simulink model "model_induction_Motor_V_F_Control_v2"  (R2017b)
settings: Solver=ode23s  StartTime=0.0  StopTime=10.0  MaxStep=1e-4  RelTol=1e-3
libraries: powerlib x20, simulink x9
settings Model: SimulationMode=accelerator  Creator=proso  LastModifiedBy=proso
settings OptimizationCC: EfficientMapNaN2IntZero=off
settings HardwareCC: TargetBitPerPointer=64  TargetBitPerSizeT=64  TargetBitPerPtrDiffT=64  TargetLongLongMode=on  TargetIntDivRoundTo=Zero  TargetEndianess=LittleEndian  TargetWordSize=64  TargetHWDeviceType=MATLAB Host  ProdEqTarget=off
settings CodeAppCC: MaxIdLength=128
settings GRTTargetCC: TargetLangStandard=C89/C90 (ANSI)  CombineOutputUpdateFcns=off  GRTInterface=on

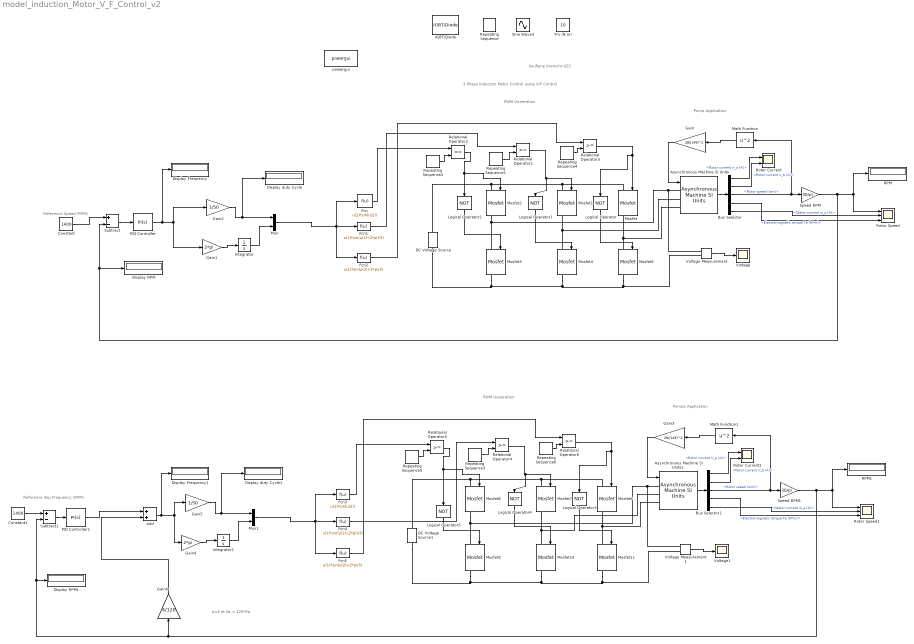
== system model_induction_Motor_V_F_Control_v2 ==
  note: p=4 et Ns = 120*f/p
  note: Reference Speed (RPM)
  note: Pump Application
  note: PWM Generation
  note: 3 Phase Induction Motor Control using V/F Control
  note: Soufiane Kremcht GE2
  note: PWM Generation
  note: Reference Slip Frequency (RPM)
  note: Pompe Application
  Add : Sum
  Asynchronous Machine SI Units : powerlib/Machines/Asynchronous Machine SI Units  RotorType=Squirrel-cage  PresetModel="15:  5.4 HP (4KW)   400 V  50Hz 1430 RPM"  MechanicalLoad=Torque Tm  ShowDetailedParameters=on  ReferenceFrame=Rotor  Units=SI  MeasurementBus=off  NominalParameters=[4000 400 50]  Stator=[1.405 0.005839]  Rotor=[1.395 0.005839]  Cage1=[1.543 0.006067]  Cage2=[3.309 0.005654]  Lm=0.1722  Mechanical=[0.0131 0.002985 2]  PolePairs=2  InitialConditions=[1 0 0 0 0 0 0 0]  SimulateSaturation=off  Saturation=[14.03593122, 27.81365428, 53.79336849, 72.68890987, 97.98006896, 148.6815601, 215.7428561, 302.9841135, 428.7778367 ; 230, 322, 414, 460, 506, 552, 598, 644, 690]  LoadFlowParameters=1492000  TsPowergui=0  TsBlock=-1  IterativeModel=Trapezoidal non iterative  IterativeDiscreteModel=Trapezoidal non iterative  Pmec=1.492e+006
  Asynchronous Machine SI Units1 : powerlib/Machines/Asynchronous Machine SI Units  RotorType=Squirrel-cage  PresetModel="15:  5.4 HP (4KW)   400 V  50Hz 1430 RPM"  MechanicalLoad=Torque Tm  ShowDetailedParameters=on  ReferenceFrame=Rotor  Units=SI  MeasurementBus=off  NominalParameters=[4000 400 50]  Stator=[1.405 0.005839]  Rotor=[1.395 0.005839]  Cage1=[1.543 0.006067]  Cage2=[3.309 0.005654]  Lm=0.1722  Mechanical=[0.0131 0.002985 2]  PolePairs=2  InitialConditions=[1 0 0 0 0 0 0 0]  SimulateSaturation=off  Saturation=[14.03593122, 27.81365428, 53.79336849, 72.68890987, 97.98006896, 148.6815601, 215.7428561, 302.9841135, 428.7778367 ; 230, 322, 414, 460, 506, 552, 598, 644, 690]  LoadFlowParameters=1492000  TsPowergui=0  TsBlock=-1  IterativeModel=Trapezoidal non iterative  IterativeDiscreteModel=Trapezoidal non iterative  Pmec=1.492e+006
  Bus Selector : BusSelector  OutputSignals=Rotor measurements.Rotor current ir_a (A),Rotor measurements.Rotor current ir_b (A),Mechanical.Rotor speed (wm),Mechanical.Electromagnetic torque Te (N*m),Stator measurements.Stator current is_a (A)
  Bus Selector1 : BusSelector  OutputSignals=Rotor measurements.Rotor current ir_a (A),Rotor measurements.Rotor current ir_b (A),Mechanical.Rotor speed (wm),Mechanical.Electromagnetic torque Te (N*m),Stator measurements.Stator current is_a (A)
  Constant : Constant  Value=1400
  Constant1 : Constant  Value=1400
  DC Voltage Source : powerlib/Electrical Sources/DC Voltage Source  Amplitude=650  Measurements=None
  DC Voltage Source1 : powerlib/Electrical Sources/DC Voltage Source  Amplitude=650  Measurements=None
  Display Frequency : Display
  Display Frequency1 : Display
  Display RPM : Display
  Display RPM1 : Display
  Display duty Cycle : Display
  Display duty Cycle1 : Display
  Fcn : Fcn  Expr=u(1)*sin(u(2))
  Fcn1 : Fcn  Expr=u(1)*sin(u(2)-(2*pi)/3)
  Fcn2 : Fcn  Expr=u(1)*sin(u(2)+2*pi/3)
  Fcn3 : Fcn  Expr=u(1)*sin(u(2))
  Fcn4 : Fcn  Expr=u(1)*sin(u(2)-(2*pi)/3)
  Fcn5 : Fcn  Expr=u(1)*sin(u(2)+2*pi/3)
  Gain : Gain  Gain=28/(149)^2
  Gain1 : Gain  Gain=2*pi
  Gain2 : Gain  Gain=1/50
  Gain3 : Gain  Gain=28/(149)^2
  Gain4 : Gain  Gain=2*pi
  Gain5 : Gain  Gain=1/50
  Gain6 : Gain  Gain=4/120
  IGBT/Diode : powerlib/Power Electronics/IGBT//Diode  Ron=1e-3  Rs=1e5  Cs=inf  Measurements=on
  Integrator : Integrator
  Integrator1 : Integrator
  Logical Operator{,1..5} (6 alike) : Logic  Operator=NOT  AllPortsSameDT=off  OutDataTypeStr=boolean
  Math Function : Math  Operator=square  SaturateOnIntegerOverflow=on
  Math Function1 : Math  Operator=square  SaturateOnIntegerOverflow=on
  Mosfet{,1..11} (12 alike) : powerlib/Power Electronics/Mosfet  Ron=0.1  Lon=0  Rd=0.01  Vfd=0  IC=0  Rs=1e5  Cs=inf  Measurements=on
  Mux : Mux  Inputs=2
  Mux1 : Mux  Inputs=2
  PID Controller : simulink/Continuous/PID Controller  Controller=PI  TimeDomain=Continuous-time  SampleTime=-1  IntegratorMethod=Forward Euler  FilterMethod=Forward Euler  Form=Parallel  UseFilter=on  ControllerParametersSource=internal  P=0.001  I=0.1  D=0  N=100  InitialConditionSource=internal  InitialConditionForIntegrator=0  InitialConditionForFilter=0  ExternalReset=none  LimitOutput=on  UpperSaturationLimit=50  LowerSaturationLimit=-50  LinearizeAsGain=on  AntiWindupMode=clamping  Kb=1  TrackingMode=off  Kt=1  PParamMin=[]  PParamMax=[]  IParamMin=[]  IParamMax=[]  DParamMin=[]  DParamMax=[]  NParamMin=[]  NParamMax=[]  KbParamMin=[]  KbParamMax=[]  KtParamMin=[]  KtParamMax=[]  POutMin=[]  POutMax=[]  IOutMin=[]  IOutMax=[]  DOutMin=[]  DOutMax=[]  NOutMin=[]  NOutMax=[]  KbOutMin=[]  KbOutMax=[]  KtOutMin=[]  KtOutMax=[]  IntegratorOutMin=[]  IntegratorOutMax=[]  FilterOutMin=[]  FilterOutMax=[]  SumOutMin=[]  SumOutMax=[]  SumI1OutMin=[]  SumI1OutMax=[]  SumI2OutMin=[]  SumI2OutMax=[]  SumI3OutMin=[]  SumI3OutMax=[]  SumDOutMin=[]  SumDOutMax=[]  SaturationOutMin=[]  SaturationOutMax=[]  IntegratorContinuousStateAttributes=''  IntegratorStateMustResolveToSignalObject=off  IntegratorRTWStateStorageClass=Auto  FilterContinuousStateAttributes=''  FilterStateMustResolveToSignalObject=off  FilterRTWStateStorageClass=Auto  DifferentiatorICPrevScaledInput=0  DifferentiatorOutMin=[]  DifferentiatorOutMax=[]  InitialConditionSetting=State (most efficient)  FilterDiffOutCoefMin=[]  FilterDiffOutCoefMax=[]  SumDenOutMin=[]  SumDenOutMax=[]  SumNumOutMin=[]  SumNumOutMax=[]  ReciprocalOutMin=[]  ReciprocalOutMax=[]  DivideOutMin=[]  DivideOutMax=[]  TunerSelectOption=Transfer Function Based (PID Tuner App)
  PID Controller1 : simulink/Continuous/PID Controller  Controller=PI  TimeDomain=Continuous-time  SampleTime=-1  IntegratorMethod=Forward Euler  FilterMethod=Forward Euler  Form=Parallel  UseFilter=on  ControllerParametersSource=internal  P=1.5  I=0.01  D=0  N=100  InitialConditionSource=internal  InitialConditionForIntegrator=0  InitialConditionForFilter=0  ExternalReset=none  LimitOutput=on  UpperSaturationLimit=50  LowerSaturationLimit=-50  LinearizeAsGain=on  AntiWindupMode=clamping  Kb=1  TrackingMode=off  Kt=1  PParamMin=[]  PParamMax=[]  IParamMin=[]  IParamMax=[]  DParamMin=[]  DParamMax=[]  NParamMin=[]  NParamMax=[]  KbParamMin=[]  KbParamMax=[]  KtParamMin=[]  KtParamMax=[]  POutMin=[]  POutMax=[]  IOutMin=[]  IOutMax=[]  DOutMin=[]  DOutMax=[]  NOutMin=[]  NOutMax=[]  KbOutMin=[]  KbOutMax=[]  KtOutMin=[]  KtOutMax=[]  IntegratorOutMin=[]  IntegratorOutMax=[]  FilterOutMin=[]  FilterOutMax=[]  SumOutMin=[]  SumOutMax=[]  SumI1OutMin=[]  SumI1OutMax=[]  SumI2OutMin=[]  SumI2OutMax=[]  SumI3OutMin=[]  SumI3OutMax=[]  SumDOutMin=[]  SumDOutMax=[]  SaturationOutMin=[]  SaturationOutMax=[]  IntegratorContinuousStateAttributes=''  IntegratorStateMustResolveToSignalObject=off  IntegratorRTWStateStorageClass=Auto  FilterContinuousStateAttributes=''  FilterStateMustResolveToSignalObject=off  FilterRTWStateStorageClass=Auto  DifferentiatorICPrevScaledInput=0  DifferentiatorOutMin=[]  DifferentiatorOutMax=[]  InitialConditionSetting=State (most efficient)  FilterDiffOutCoefMin=[]  FilterDiffOutCoefMax=[]  SumDenOutMin=[]  SumDenOutMax=[]  SumNumOutMin=[]  SumNumOutMax=[]  ReciprocalOutMin=[]  ReciprocalOutMax=[]  DivideOutMin=[]  DivideOutMax=[]  TunerSelectOption=Transfer Function Based (PID Tuner App)
  RPM : Display
  RPM1 : Display
  Relational Operator{1..6} (6 alike) : RelationalOperator  OutDataTypeStr=boolean  RndMeth=Simplest
  Repeating Sequence : simulink/Sources/Repeating Sequence  rep_seq_t=[0 .1 10]  rep_seq_y=[0 50 50]
  Repeating Sequence{1..6} (6 alike) : simulink/Sources/Repeating Sequence  rep_seq_t="[0 (1/5000)/4  (1/5000)/2 (3/5000)/4 1/5000]"  rep_seq_y=[0 1 0 -1 0]
  Rotor Current : Scope  NumInputPorts=2
  Rotor Current1 : Scope  NumInputPorts=2
  Rotor Speed : Scope  NumInputPorts=3
  Rotor Speed1 : Scope  NumInputPorts=3
  Sine Wave3 : Sin  Amplitude=0.9  Frequency=100*pi  SampleTime=0
  Speed RPM : Gain  Gain=30/pi
  Speed RPM1 : Gain  Gain=30/pi
  Subtract : Sum  Inputs=+-
  Subtract1 : Sum  Inputs=+-
  Tm (N.m) : Constant  Value=10
  Voltage : Scope
  Voltage Measurement : powerlib/Measurements/Voltage Measurement  PhasorSimulation=off  OutputType=Complex  PSBequivalent=0
  Voltage Measurement1 : powerlib/Measurements/Voltage Measurement  PhasorSimulation=off  OutputType=Complex  PSBequivalent=0
  Voltage1 : Scope
  powergui : powerlib/powergui  Priority=1  SimulationMode=Discrete  SampleTime=1e-5  frequency=60  Iterations=50  frequencyindice=0  Pbase=100e6  ErrMax=1e-4  UnitsV=kV  UnitsW=MW  buscounter=0  FunctionMessages=off  echomessages=off  EnableUseOfTLC=off  CurrentSourceSwitches=off  DisableSnubberDevices=off  DisableRonSwitches=off  DisableVfSwitches=off  DisplayEquations=off  SolverType=Tustin/Backward Euler (TBE)  Interpol=off  ExternalGateDelay=off  methode=off  Ts=100  x0status=blocks  SPID=on  SwTol=0  HookPort=off  RestoreLinks=warning  ResistiveCurrentMeasurement=off  Frange=[0:2:500]  Ylog=off  Xlog=on  ShowGrid=off  save=off  variable=ZData  structure=0  ZoomFFT=off  StartTime=0.0  cycles=1  DisplayStyle=1  fundamental=60  FreqAxis=off  MaxFrequency=1000  frequencyindicesteady=1  RmsSteady=1  display=off
  wires:
  Gain2/1 -> Display duty Cycle/1, Mux/1
  Bus Selector/3 -> Math Function/1, Speed RPM/1  "<Rotor speed (wm)>"
  Bus Selector/1 -> Rotor Current/1  "<Rotor current ir_a (A)>"
  Bus Selector/4 -> Rotor Speed/3  "<Electromagnetic torque Te (N*m)>"
  Bus Selector/2 -> Rotor Current/2  "<Rotor current ir_b (A)>"
  Asynchronous Machine SI Units/1 -> Bus Selector/1
  Voltage Measurement/1 -> Voltage/1
  Gain1/1 -> Integrator/1
  Integrator/1 -> Mux/2
  Speed RPM/1 -> Subtract/2, Display RPM/1, Rotor Speed/1, RPM/1
  Mux/1 -> Fcn/1, Fcn2/1, Fcn1/1
  Relational Operator3/1 -> Mosfet/1, Logical Operator/1
  Logical Operator/1 -> Mosfet5/1
  Logical Operator2/1 -> Mosfet3/1
  Logical Operator1/1 -> Mosfet4/1
  Bus Selector/5 -> Rotor Speed/2  "<Stator current is_a (A)>"
  Constant/1 -> Subtract/1
  Subtract/1 -> PID Controller/1
  PID Controller/1 -> Display Frequency/1, Gain1/1, Gain2/1
  Math Function/1 -> Gain/1
  Repeating Sequence4/1 -> Relational Operator3/2
  Repeating Sequence1/1 -> Relational Operator1/2
  Repeating Sequence2/1 -> Relational Operator2/2
  Relational Operator2/1 -> Mosfet2/1, Logical Operator2/1
  Relational Operator1/1 -> Mosfet1/1, Logical Operator1/1
  Gain/1 -> Asynchronous Machine SI Units/1
  Fcn/1 -> Relational Operator2/1
  Fcn2/1 -> Relational Operator3/1
  Fcn1/1 -> Relational Operator1/1
  Fcn3/1 -> Relational Operator5/1
  Fcn5/1 -> Relational Operator6/1
  Fcn4/1 -> Relational Operator4/1
  Math Function1/1 -> Gain3/1
  Subtract1/1 -> PID Controller1/1
  Relational Operator6/1 -> Mosfet6/1, Logical Operator3/1
  Repeating Sequence5/1 -> Relational Operator5/2
  Integrator1/1 -> Mux1/2
  Bus Selector1/5 -> Rotor Speed1/2  "<Stator current is_a (A)>"
  Relational Operator5/1 -> Mosfet8/1, Logical Operator5/1
  Bus Selector1/2 -> Rotor Current1/2  "<Rotor current ir_b (A)>"
  Speed RPM1/1 -> Gain6/1, Display RPM1/1, Subtract1/2, Rotor Speed1/1, RPM1/1
  Repeating Sequence6/1 -> Relational Operator6/2
  Constant1/1 -> Subtract1/1
  Bus Selector1/3 -> Math Function1/1, Speed RPM1/1  "<Rotor speed (wm)>"
  Repeating Sequence3/1 -> Relational Operator4/2
  Logical Operator4/1 -> Mosfet10/1
  Logical Operator5/1 -> Mosfet9/1
  Voltage Measurement1/1 -> Voltage1/1
  Gain3/1 -> Asynchronous Machine SI Units1/1
  Mux1/1 -> Fcn3/1, Fcn5/1, Fcn4/1
  Asynchronous Machine SI Units1/1 -> Bus Selector1/1
  Bus Selector1/4 -> Rotor Speed1/3  "<Electromagnetic torque Te (N*m)>"
  Gain4/1 -> Integrator1/1
  Gain5/1 -> Display duty Cycle1/1, Mux1/1
  Relational Operator4/1 -> Mosfet7/1, Logical Operator4/1
  Bus Selector1/1 -> Rotor Current1/1  "<Rotor current ir_a (A)>"
  Logical Operator3/1 -> Mosfet11/1
  Gain6/1 -> Add/2
  PID Controller1/1 -> Add/1
  Add/1 -> Display Frequency1/1, Gain4/1, Gain5/1
  connections:
  Asynchronous Machine SI Units/LConn3 -- Mosfet/RConn1 -- Mosfet5/LConn1
  DC Voltage Source/LConn1 -- Mosfet3/RConn1 -- Mosfet4/RConn1 -- Mosfet5/RConn1 -- Voltage Measurement/LConn2
  Asynchronous Machine SI Units/LConn2 -- Mosfet4/LConn1 -- Mosfet1/RConn1
  Asynchronous Machine SI Units/LConn1 -- Voltage Measurement/LConn1 -- Mosfet3/LConn1 -- Mosfet2/RConn1
  DC Voltage Source/RConn1 -- Mosfet2/LConn1 -- Mosfet1/LConn1 -- Mosfet/LConn1
  Mosfet6/LConn1 -- DC Voltage Source1/RConn1 -- Mosfet8/LConn1 -- Mosfet7/LConn1
  Mosfet8/RConn1 -- Mosfet9/LConn1 -- Asynchronous Machine SI Units1/LConn1 -- Voltage Measurement1/LConn1
  Voltage Measurement1/LConn2 -- DC Voltage Source1/LConn1 -- Mosfet9/RConn1 -- Mosfet10/RConn1 -- Mosfet11/RConn1
  Mosfet6/RConn1 -- Asynchronous Machine SI Units1/LConn3 -- Mosfet11/LConn1
  Mosfet7/RConn1 -- Asynchronous Machine SI Units1/LConn2 -- Mosfet10/LConn1
